simulink model "Mission_1"  (R2019a)
settings: Solver=FixedStepAuto  StartTime=0.0  StopTime=100  FixedStep=0.2  RelTol=1e-3
libraries: Lib_Solve_ModelSource_TMATS x2
settings Model: Creator=anton  LastModifiedBy=anton

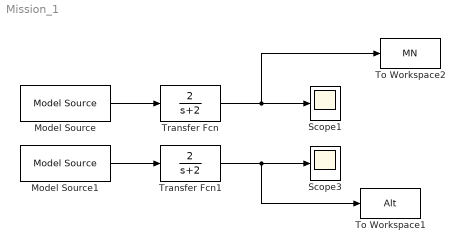
== system Mission_1 ==
  Model Source : Lib_Solve_ModelSource_TMATS/Model Source  T_vec_M=[0 5 10 30 70 100]  input_array_M=[0 0 0.6 0.4 0.3 0.3]
  Model Source1 : Lib_Solve_ModelSource_TMATS/Model Source  T_vec_M=[0 5 10 30 70 100]  input_array_M=[0 0 500 550 480 400]
  Scope1 : Scope
  Scope3 : Scope
  To Workspace1 : ToWorkspace  VariableName=Alt  SaveFormat=Timeseries  SampleTime=-1
  To Workspace2 : ToWorkspace  VariableName=MN  SaveFormat=Timeseries  SampleTime=-1
  Transfer Fcn : TransferFcn  Numerator=2  Denominator=[1 2]
  Transfer Fcn1 : TransferFcn  Numerator=2  Denominator=[1 2]
  wires:
  Model Source/1 -> Transfer Fcn/1
  Transfer Fcn/1 -> To Workspace2/1, Scope1/1
  Transfer Fcn1/1 -> To Workspace1/1, Scope3/1
  Model Source1/1 -> Transfer Fcn1/1
